simulink model "integrated_campus"  (Simulink 8.1)
settings: Solver=ode3  SolverMode=SingleTasking  StartTime=0.0  StopTime=24*3600  FixedStep=5  MaxStep=1/60  RelTol=1e-3
InitFcn:
  | Ts=1e-4; Tpv = 0.1;
undefined symbols (not defined in the file or in its folder): D11, Delta
libraries: powerlib x41, CampusEnergyModeling x37, powerlib_meascontrol x11, simulink x7
(part 2 of 2)

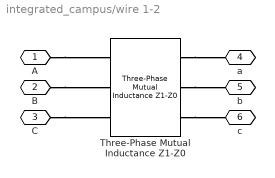
== system integrated_campus/wire 1-2 ==
  Three-Phase Mutual Inductance Z1-Z0 : powerlib/Elements/Three-Phase Mutual Inductance Z1-Z0  LConnTagsString=a|b|c  RConnTagsString=A|B|C  PositiveSequence=[R1 X1/376.9911]*L/1000  ZeroSequence=[R0 X0/376.9911]*L/1000
  A : PMIOPort  Port=1  Side=Left
  B : PMIOPort  Port=2  Side=Left
  "C " : PMIOPort  Port=3  Side=Left
  a : PMIOPort  Port=4  Side=Right
  b : PMIOPort  Port=5  Side=Right
  c : PMIOPort  Port=6  Side=Right
  connections:
  Three-Phase Mutual Inductance Z1-Z0/RConn3 -- c/RConn1
  Three-Phase Mutual Inductance Z1-Z0/RConn2 -- b/RConn1
  Three-Phase Mutual Inductance Z1-Z0/RConn1 -- a/RConn1
  "C "/RConn1 -- Three-Phase Mutual Inductance Z1-Z0/LConn3
  B/RConn1 -- Three-Phase Mutual Inductance Z1-Z0/LConn2
  A/RConn1 -- Three-Phase Mutual Inductance Z1-Z0/LConn1

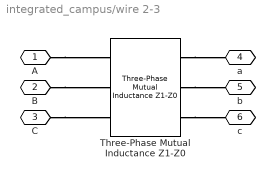
== system integrated_campus/wire 2-3 ==
  Three-Phase Mutual Inductance Z1-Z0 : powerlib/Elements/Three-Phase Mutual Inductance Z1-Z0  LConnTagsString=a|b|c  RConnTagsString=A|B|C  PositiveSequence=[R1 X1/376.9911]*L/1000  ZeroSequence=[R0 X0/376.9911]*L/1000
  A : PMIOPort  Port=1  Side=Left
  B : PMIOPort  Port=2  Side=Left
  "C " : PMIOPort  Port=3  Side=Left
  a : PMIOPort  Port=4  Side=Right
  b : PMIOPort  Port=5  Side=Right
  c : PMIOPort  Port=6  Side=Right
  connections:
  A/RConn1 -- Three-Phase Mutual Inductance Z1-Z0/LConn1
  B/RConn1 -- Three-Phase Mutual Inductance Z1-Z0/LConn2
  "C "/RConn1 -- Three-Phase Mutual Inductance Z1-Z0/LConn3
  Three-Phase Mutual Inductance Z1-Z0/RConn1 -- a/RConn1
  Three-Phase Mutual Inductance Z1-Z0/RConn2 -- b/RConn1
  Three-Phase Mutual Inductance Z1-Z0/RConn3 -- c/RConn1

== system integrated_campus/wire 4-5 ==
  Three-Phase Mutual Inductance Z1-Z0 : powerlib/Elements/Three-Phase Mutual Inductance Z1-Z0  LConnTagsString=a|b|c  RConnTagsString=A|B|C  PositiveSequence=[R1 X1/376.9911]*L/1000  ZeroSequence=[R0 X0/376.9911]*L/1000
  A : PMIOPort  Port=1  Side=Left
  B : PMIOPort  Port=2  Side=Left
  "C " : PMIOPort  Port=3  Side=Left
  a : PMIOPort  Port=4  Side=Right
  b : PMIOPort  Port=5  Side=Right
  c : PMIOPort  Port=6  Side=Right
  connections:
  A/RConn1 -- Three-Phase Mutual Inductance Z1-Z0/LConn1
  B/RConn1 -- Three-Phase Mutual Inductance Z1-Z0/LConn2
  "C "/RConn1 -- Three-Phase Mutual Inductance Z1-Z0/LConn3
  Three-Phase Mutual Inductance Z1-Z0/RConn1 -- a/RConn1
  Three-Phase Mutual Inductance Z1-Z0/RConn2 -- b/RConn1
  Three-Phase Mutual Inductance Z1-Z0/RConn3 -- c/RConn1

== matlab function Campus Thermal Model/PrepOutputs1 ==
  data: u input double; Temp output double; Input output double; InOutTemp output double; Pow output double; PPD output double
function [Temp,Input,InOutTemp, Pow, PPD] = fcn(u)

Temp = u(1:7);          % Out, Room Temp
Input = u(8:9);         % Flow Rate, Load 
InOutTemp = u(10:11);   % Inlet/Outlet Water Temperature
Pow = u(12:13);         % Power
PPD = u(14);            % Percentage of People Dissatisfied [%]

== matlab function Campus Thermal Model/PrepOutputs ==
  data: u input double; Temp output double; ChilPow output double; ChilTemp output double; MaxChilFlow output double; Input01 output double; Input02 output double; InOutTemp output double; PumpPow output double
function [Temp,ChilPow,ChilTemp, MaxChilFlow, Input01, Input02, InOutTemp, PumpPow] = fcn(u)

Temp = u(1);        % Temperature(Outdoor, Zones)
ChilPow = u(2);     % Chiller Power
ChilTemp = u(3);    % Chiller Water Temperature
MaxChilFlow = u(4); % Maximum Chiller Flow 
Input01 = u(5:6);   % Mass Flow Rate and Power Load 
Input02 = u(7:8);   % Mass Flow Rate and Power Load
InOutTemp = u(9:12);% Inlet/Outlet Water Temperature   
PumpPow = u(13);    % Pump Power

== matlab function Campus Supervisory Control/Control Function ==
  data: Inputs output double; Campus_Outputs input double; Weather input double; Time input double; Price input double; Signal input double; Thresh input double
function Inputs = fcn(Campus_Outputs, Weather, Time, Price, Signal, Thresh)
%% CONTROL LOOP FOR BUILDING
lights = Signal(1);
chiller = Signal(2);
room = Signal(3);
plant = Signal(4);

%% Lights Schedule
if Time < 8
    LightsSch1 = 0.1;
    LightsSch2 = 0.1;
elseif Time < 9
    LightsSch1 = 0.9;
    LightsSch2 = 0.9;
elseif Time < 10
    LightsSch1 = 0.95;
    LightsSch2 = 0.95;
elseif Time < 11
    LightsSch1 = 1;
    LightsSch2 = 1;
elseif Time < 12
    LightsSch1 = 0.95;
    LightsSch2 = 0.95;
elseif Time < 13
    LightsSch1 = 0.8;
    LightsSch2 = 0.8;
elseif Time < 14
    LightsSch1 = 0.9;
    LightsSch2 = 0.9;
elseif Time < 18
    LightsSch1 = 1;
    LightsSch2 = 1;
elseif Time < 19
    LightsSch1 = 0.6;
    LightsSch2 = 0.6;
elseif Time < 21
    LightsSch1 = 0.2;
    LightsSch2 = 0.2;
else
    LightsSch1 = 0.05;
    LightsSch2 = 0.05;
end

%% CONTROL
ChilledWaterSetpoint = 7.22;
Room1CoolingSetpoint = 21;
Room2CoolingSetpoint = 21;
Room1HeatingSetpoint = 20;
Room2HeatingSetpoint = 20;
PlantAct = 1;
%% Lights
if lights == 1
    LightsFactor = 1;
    if Price > Thresh(1)
        LightsFactor = 1 - (Price-Thresh(1))*20;
    end
    LightsSch1 = LightsSch1*LightsFactor;
    LightsSch2 = LightsSch2*LightsFactor;
end
%% Chiller
if chiller == 1
    if Price > Thresh(2)
        ChilledWaterSetpoint = 7.22 + (Price-Thresh(2))*400;
    end
end
%% Room Setpoints
if room == 1
    if Price > Thresh(3)
        Room1CoolingSetpoint = 22 + (Price-Thresh(3))*500;
        Room2CoolingSetpoint = 22 + (Price-Thresh(3))*500;
        Room1HeatingSetpoint = 20;
        Room2HeatingSetpoint = 20;
    end
end
%% Plant
if plant == 1
    PlantAct = 1;
    if Price > Thresh(4)
        PlantAct = 0;
    end
end
%% SET OUTPUTS
Inputs = [ChilledWaterSetpoint,...
    Room1CoolingSetpoint,...
    Room2CoolingSetpoint,...
    Room1HeatingSetpoint,...
    Room2HeatingSetpoint,...
    PlantAct,...
    LightsSch1,...
    LightsSch2];

== matlab function Campus Thermal Model/PrepOutputs3 ==
  data: MaxMassFlow1 output double; MaxFlow input double; MaxMassFlow2 output double
function [MaxMassFlow1, MaxMassFlow2] = fcn(MaxFlow)
% Transform into [Kg/s] Split Evenly
MaxFlow = MaxFlow*1000;
%if Input1+Input2 > MaxFlow
MaxMassFlow1 = MaxFlow/2;
MaxMassFlow2 = MaxFlow/2;
%else
%    MaxMassFlow1 =  
%    MaxMassFlow2 = MaxFlow - Input;
%end

== matlab function Campus Thermal Model/PrepOutputs4 ==
  data: u input double; Temp output double; Input output double; InOutTemp output double; Pow output double
function [Temp,Input,InOutTemp,Pow] = fcn(u)

Temp = u(1:7);          % Out, Room Temp
Input = u(8:9);         % Flow Rate, Load 
InOutTemp = u(10:11);   % Inlet/Outlet Water Temperature
Pow = u(12:13);         % Total Power

== matlab function Campus Supervisory Control/Display Power ==
  data: Scenario output double; Baseline input double; y output double; Actual input double; Price input double
function [Scenario, y] = fcn(Baseline, Actual, Price)
%#codegen

% Total Power Consumption
y1 = sum(Actual(1:end-1));
y2 = sum(Baseline(1:end-1));

% Plant Power Consumption
y3 = sum(Actual([5 6]));
y4 = sum(Baseline([5 6]));

% Building 1 Power Consumption
y5 = sum(Actual([1 2]));
y6 = sum(Baseline([1 2]));

% Building 2 Power Consumption
y7 = sum(Actual([3 4]));
y8 = sum(Baseline([3 4]));

% Energy Cost
y9 = y1*Price/1000;
y10 = y2*Price/1000;

% Percentage of People Dissatisfied (PPD)
y11 = Actual(7);
y12 = Baseline(7);

% Put Together
y = [y1 y2 y3 y4 y5 y6 y7 y8 y9 y10 y11 y12];

% Baseline
Scenario = Actual;

== matlab function Campus Thermal Model/PrepOutputs6 ==
  data: Input1 input double; Input2 input double; mflow1 output double; pow1 output double; mflow2 output double; pow2 output double
function [mflow1, pow1, mflow2, pow2] = fcn(Input1, Input2)
ratio = 0.005;
mflow1 = Input1(1)/ratio/1000;
pow1 = Input1(2);
mflow2 = Input2(1)/ratio/1000; 
pow2 = Input2(2);
